simulink model "openloop_SASA_original"  (R2016a)
settings: Solver=ode3  StartTime=0.0  StopTime=4  FixedStep=1e-5  RelTol=1e-3
values from neighbouring files (symbols this model uses):
  A = zeros(modes,modes)    [matrice_two_piezo.m]
  B = zeros(modes,modes)    [matrice_two_piezo.m]
  C = zeros(1,modes)    [matrice_two_piezo.m]
  E = zeros(modes,modes)    [matrice_two_piezo.m]
  Q = double(Q)    [matrice_two_piezo.m]
settings Model: Creator=yashwanth  LastModifiedBy=yash9
settings DataIOCC: LimitDataPoints=on
settings DebuggingCC: AllowSymbolicDim=off
settings ModelReferenceCC: PropagateSignalLabelsOutOfModel=off
settings GRTTargetCC: GeneratePreprocessorConditionals=Use local settings

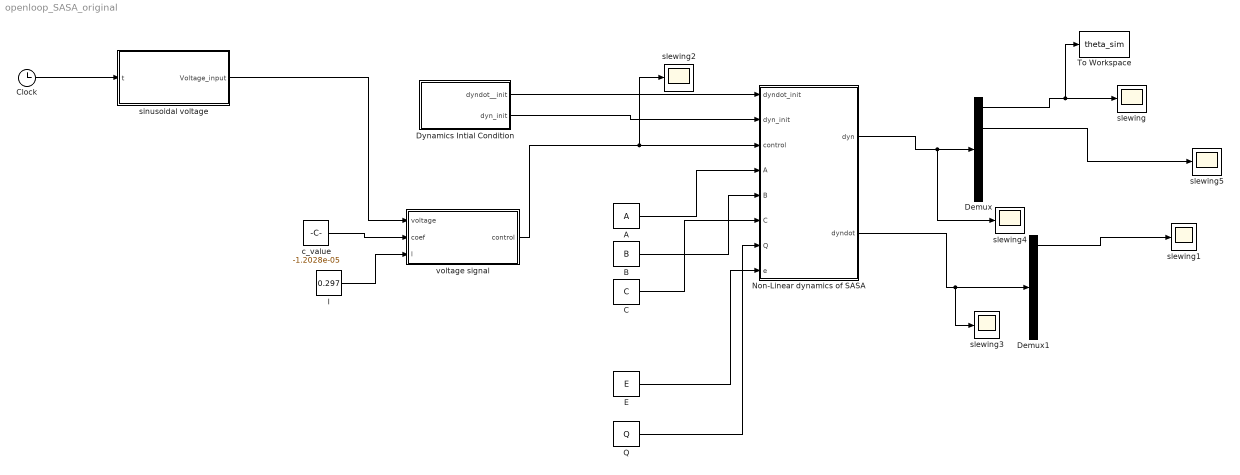
== system openloop_SASA_original ==
  " Non-Linear dynamics of SASA" : Subsystem
  A : Constant  Value=A  VectorParams1D=off
  B : Constant  Value=B  VectorParams1D=off
  C : Constant  Value=C  VectorParams1D=off
  Clock : Clock
  Demux : Demux  Outputs=5
  Demux1 : Demux  Outputs=5
  Dynamics Intial Condition : Subsystem
  E : Constant  Value=E  VectorParams1D=off
  Q : Constant  Value=Q
  To Workspace : ToWorkspace  VariableName=theta_sim  SaveFormat=Timeseries  SampleTime=-1
  c_value : Constant  Value=-1.2028e-05
  l : Constant  Value=0.297
  sinusoidal voltage : MATLAB Function  TreatAsAtomicUnit=on
  slewing{,1..5} (6 alike) : Scope
  voltage signal : MATLAB Function  TreatAsAtomicUnit=on
  wires:
  Dynamics Intial Condition/2(dyn_init) -> " Non-Linear dynamics of SASA"/2(dyn_init)
  Dynamics Intial Condition/1(dyndot__init) -> " Non-Linear dynamics of SASA"/1(dyndot_init)
  " Non-Linear dynamics of SASA"/1(dyn) -> slewing4/1, Demux/1
  Demux1/1 -> slewing1/1
  " Non-Linear dynamics of SASA"/2(dyndot) -> slewing3/1, Demux1/1
  voltage signal/1(control) -> slewing2/1, " Non-Linear dynamics of SASA"/3(control)
  c_value/1 -> voltage signal/2(coef)
  l/1 -> voltage signal/3(l)
  sinusoidal voltage/1(Voltage_input) -> voltage signal/1(voltage)
  Demux/1 -> To Workspace/1, slewing/1
  A/1 -> " Non-Linear dynamics of SASA"/4(A)
  B/1 -> " Non-Linear dynamics of SASA"/5(B)
  C/1 -> " Non-Linear dynamics of SASA"/6(C)
  E/1 -> " Non-Linear dynamics of SASA"/8(e)
  Q/1 -> " Non-Linear dynamics of SASA"/7(Q)
  Clock/1 -> sinusoidal voltage/1(t)
  Demux/2 -> slewing5/1

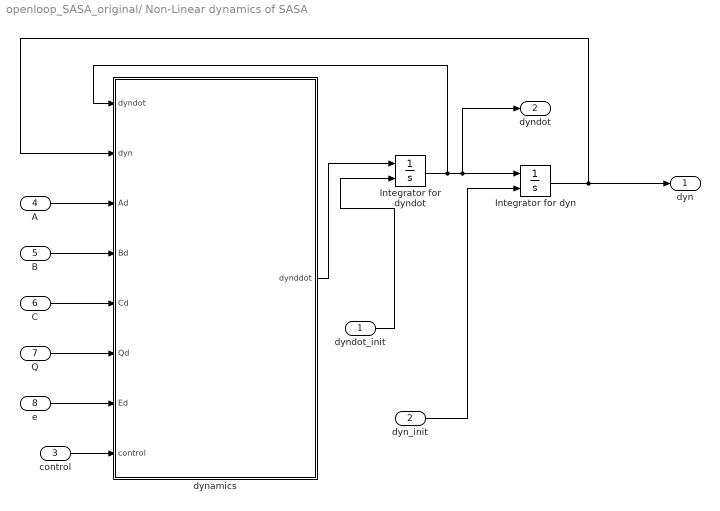
== system openloop_SASA_original/ Non-Linear dynamics of SASA ==
  dyndot_init : Inport
  dyn_init : Inport  Port=2
  control : Inport  Port=3
  A : Inport  Port=4
  B : Inport  Port=5
  C : Inport  Port=6
  Q : Inport  Port=7
  e : Inport  Port=8
  Integrator for dyn : Integrator  InitialConditionSource=external  InitialCondition=-0.1  AbsoluteTolerance=1e-3
  Integrator for dyndot : Integrator  InitialConditionSource=external  InitialCondition=-0.1  UpperSaturationLimit=1e20  LowerSaturationLimit=-1e20  AbsoluteTolerance=1e-10
  dynamics : MATLAB Function  TreatAsAtomicUnit=on
  dyn : Outport
  dyndot : Outport  Port=2
  wires:
  Integrator for dyndot/1 -> dyndot/1, Integrator for dyn/1, dynamics/1(dyndot)
  Integrator for dyn/1 -> dyn/1, dynamics/2(dyn)
  dyndot_init/1 -> Integrator for dyndot/2
  dyn_init/1 -> Integrator for dyn/2
  control/1 -> dynamics/8(control)
  A/1 -> dynamics/3(Ad)
  B/1 -> dynamics/4(Bd)
  C/1 -> dynamics/5(Cd)
  Q/1 -> dynamics/6(Qd)
  e/1 -> dynamics/7(Ed)
  dynamics/1(dynddot) -> Integrator for dyndot/1

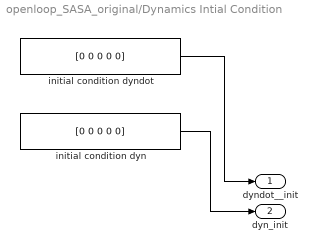
== system openloop_SASA_original/Dynamics Intial Condition ==
  initial condition dyn : Constant  Value=[0 0 0 0 0]
  initial condition dyndot : Constant  Value=[0 0 0 0 0]
  dyndot__init : Outport
  dyn_init : Outport  Port=2
  wires:
  initial condition dyn/1 -> dyn_init/1
  initial condition dyndot/1 -> dyndot__init/1

== matlab function openloop_SASA_original/ Non-Linear dynamics of SASA/dynamics ==
  data: dyndot input; dyn input; dynddot output; Ad input; Bd input; Cd input; Qd input; Ed input; control input
function dynddot  = fcn(dyndot,dyn,Ad,Bd,Cd,Qd,Ed,control)
%#codegen
% function dynamics of spacecraft and the rightSA
% generating matrices to use in the dynamics.
% number of modes used =4 (we use 2nd order equations here)
%dynamics of theta and eta
dyndot1=dyndot(1);
dyndot2=[dyndot(2);dyndot(3);dyndot(4);dyndot(5)];
dyn2=[dyn(2);dyn(3);dyn(4);dyn(5)];
AA= [Qd+2*(transpose(dyn2)*(Ad-Bd)*dyn2) 2*Cd;2*Cd' 2*Ad];

B1= [2*((dyndot1*dyndot2'*(Ad-Bd)*dyn2) + (dyn2'*(Ad-Bd)*dyndot1*dyndot2)) + 0.01*dyndot1 + 0.01*dyn(1) ;2*((-(Ad-Bd)*(dyndot1^2)*dyn2)+ (Ed*(dyn2+0.01*dyndot2)))];

dynddot= inv(AA)*(-B1+[0;2*control]);

== matlab function openloop_SASA_original/sinusoidal voltage ==
  data: t input; Voltage_input output
function Voltage_input = fcn(t)

Voltage_input=[40*sin(2*pi*1*t);0];

== matlab function openloop_SASA_original/voltage signal ==
  data: voltage input; control output; coef input; l input
function control = fcn(voltage,coef,l)

c=-coef;

lp=7.244*10^-2; % length of the piezo
% Piezo1 location 
lp_1=1.2*10^-2; % distance of the root of the piezo from that beamroot
lp_2=lp_1+lp;
% distance between Piezo 1 and Piezo 2 
dpp=4.7*10^-3;
lp1_1= lp_2+dpp;
lp1_2= lp1_1+lp;


phi1_l1=(pi^2*lp_1)/(l^2) +pi/l* sin((pi*lp_1)/l);
phi2_l1=  - 2*(2*pi^2*lp_1)/l^2 +(2*pi/l)*sin((2*pi*lp_1)/l);
phi3_l1=(9*pi^2*lp_1)/(l^2) +(3*pi)/l*sin((3*pi*lp_1)/l) ;
phi4_l1=-2*(8*pi^2*lp_1)/l^2 +(4*pi)/l*sin((4*pi*lp_1)/l);

phi1_l2=(pi^2*lp_2)/(l^2) +pi/l* sin((pi*lp_2)/l);
phi2_l2=  - 2*(2*pi^2*lp_2)/l^2 +(2*pi/l)*sin((2*pi*lp_2)/l);
phi3_l2=(9*pi^2*lp_2)/(l^2) +(3*pi)/l*sin((3*pi*lp_2)/l) ;
phi4_l2=-2*(8*pi^2*lp_2)/l^2 +(4*pi)/l*sin((4*pi*lp_2)/l);

phi1_l3=(pi^2*lp1_1)/(l^2) +pi/l* sin((pi*lp1_1)/l);
phi2_l3=  - 2*(2*pi^2*lp1_1)/l^2 +(2*pi/l)*sin((2*pi*lp1_1)/l);
phi3_l3=(9*pi^2*lp1_1)/(l^2) +(3*pi)/l*sin((3*pi*lp1_1)/l) ;
phi4_l3=-2*(8*pi^2*lp1_1)/l^2 +(4*pi)/l*sin((4*pi*lp1_1)/l);

phi1_l4=(pi^2*lp1_2)/(l^2) +pi/l* sin((pi*lp1_2)/l);
phi2_l4=  - 2*(2*pi^2*lp1_2)/l^2 +(2*pi/l)*sin((2*pi*lp1_2)/l);
phi3_l4=(9*pi^2*lp1_2)/(l^2) +(3*pi)/l*sin((3*pi*lp1_2)/l) ;
phi4_l4=-2*(8*pi^2*lp1_2)/l^2 +(4*pi)/l*sin((4*pi*lp1_2)/l);

control= c*[phi1_l2-phi1_l1 phi1_l4-phi1_l3;phi2_l2-phi2_l1 phi2_l4-phi2_l3;phi3_l2-phi3_l1 phi3_l4-phi3_l3;phi4_l2-phi4_l1 phi4_l4-phi4_l3]*voltage;
%Voltage= pinv([phi1_l2-phi1_l1 phi1_l4-phi1_l3;phi2_l2-phi2_l1 phi2_l4-phi2_l3;phi3_l2-phi3_l1 phi3_l4-phi3_l3;phi4_l2-phi4_l1 phi4_l4-phi4_l3])*control/c;
